simulink model "RadioComm2015"  (Simulink 8.1)
settings: Solver=ode45  StartTime=0.0  StopTime=10.0  RelTol=1e-3
libraries: simulink x6
settings Model: Creator=Brian  LastModifiedBy=Brian
settings DataIOCC: SignalLoggingSaveFormat=Dataset
settings OptimizationCC: ExpressionDepthLimit=128
settings DebuggingCC: FcnCallInpInsideContextMsg=EnableAllAsError
settings GRTTargetCC: CombineOutputUpdateFcns=on  GRTInterface=off

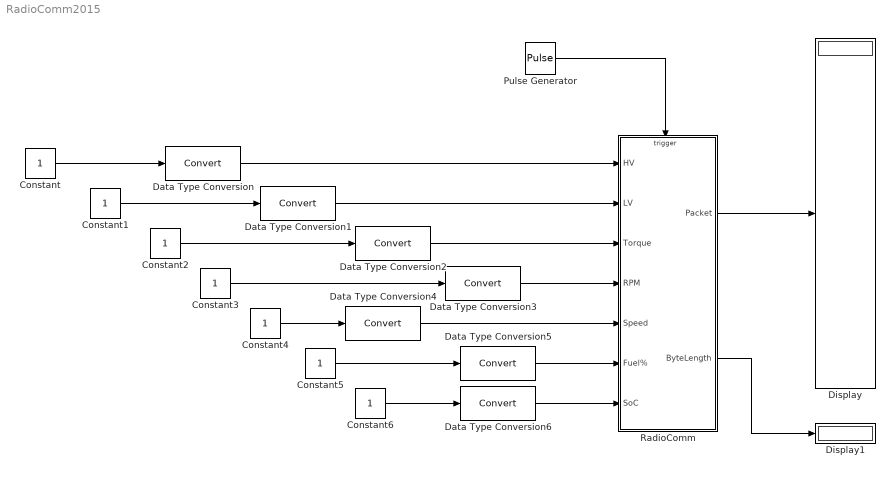
== system RadioComm2015 ==
  Constant{,1..6} (7 alike) : Constant
  Data Type Conversion{,1..6} (7 alike) : DataTypeConversion
  Display : Display
      settings: Format=hex (Stored Integer)
  Display1 : Display
      settings: Format=decimal (Stored Integer)
  Pulse Generator : DiscretePulseGenerator  PulseType=Time based  Period=.5  PulseWidth=5
  RadioComm : Subsystem
  wires:
  Constant/1 -> Data Type Conversion/1
  Constant1/1 -> Data Type Conversion1/1
  Constant2/1 -> Data Type Conversion2/1
  Constant3/1 -> Data Type Conversion3/1
  Constant4/1 -> Data Type Conversion4/1
  Constant5/1 -> Data Type Conversion5/1
  Constant6/1 -> Data Type Conversion6/1
  RadioComm/1(Packet) -> Display/1
  Data Type Conversion/1 -> RadioComm/1(HV)
  Data Type Conversion1/1 -> RadioComm/2(LV)
  Data Type Conversion2/1 -> RadioComm/3(Torque)
  Data Type Conversion3/1 -> RadioComm/4(RPM)
  Data Type Conversion4/1 -> RadioComm/5(Speed)
  Data Type Conversion5/1 -> RadioComm/6(Fuel%)
  Data Type Conversion6/1 -> RadioComm/7(SoC)
  RadioComm/2(ByteLength) -> Display1/1
  Pulse Generator/1 -> RadioComm/Trigger

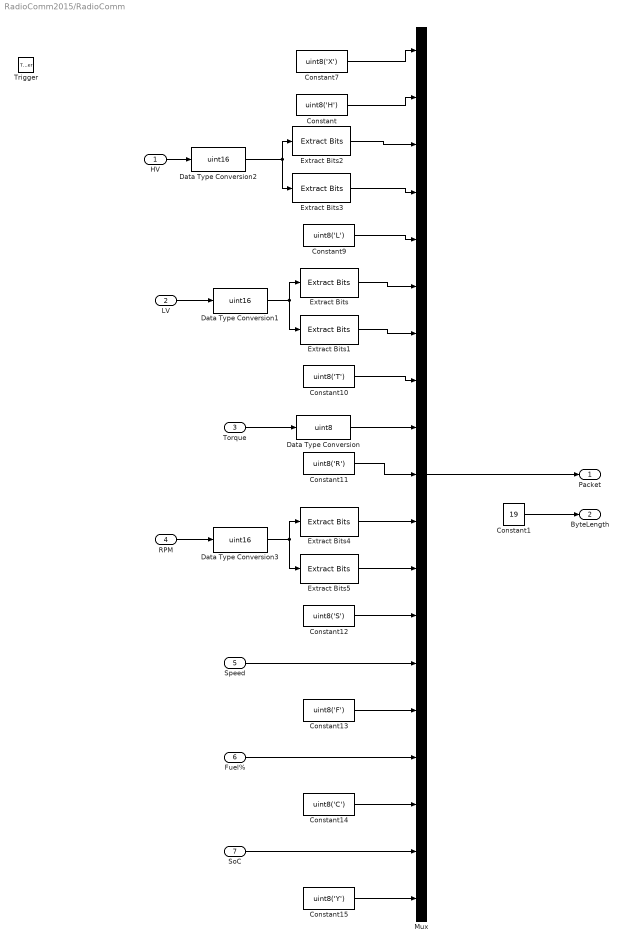
== system RadioComm2015/RadioComm ==
  HV : Inport  OutDataTypeStr=single
  LV : Inport  Port=2  OutDataTypeStr=single
  Torque : Inport  Port=3  OutDataTypeStr=int8
  RPM : Inport  Port=4  OutDataTypeStr=uint16
  Speed : Inport  Port=5  OutDataTypeStr=uint8
  Fuel% : Inport  Port=6  OutDataTypeStr=uint8
  SoC : Inport  Port=7  OutDataTypeStr=uint8
  Trigger : TriggerPort  PortDimensions=1
  Constant : Constant  Value=uint8('H')  OutDataTypeStr=uint8
  Constant1 : Constant  Value=19  OutDataTypeStr=uint8
  Constant10 : Constant  Value=uint8('T')  OutDataTypeStr=uint8
  Constant11 : Constant  Value=uint8('R')  OutDataTypeStr=uint8
  Constant12 : Constant  Value=uint8('S')  OutDataTypeStr=uint8
  Constant13 : Constant  Value=uint8('F')  OutDataTypeStr=uint8
  Constant14 : Constant  Value=uint8('C')  OutDataTypeStr=uint8
  Constant15 : Constant  Value=uint8('Y')  OutDataTypeStr=uint8
  Constant7 : Constant  Value=uint8('X')  OutDataTypeStr=uint8
  Constant9 : Constant  Value=uint8('L')  OutDataTypeStr=uint8
  Data Type Conversion : DataTypeConversion  OutDataTypeStr=uint8  ConvertRealWorld=Stored Integer (SI)  LockScale=on
  Data Type Conversion1 : DataTypeConversion  OutDataTypeStr=uint16  ConvertRealWorld=Stored Integer (SI)  LockScale=on
  Data Type Conversion2 : DataTypeConversion  OutDataTypeStr=uint16  ConvertRealWorld=Stored Integer (SI)  LockScale=on
  Data Type Conversion3 : DataTypeConversion  OutDataTypeStr=uint16  ConvertRealWorld=Stored Integer (SI)  LockScale=on
  Extract Bits : simulink/Logic and Bit Operations/Extract Bits  bitsToExtract=Upper half  numBits=8  bitIdxRange=[0 7]  outScalingMode=Treat bit field as an integer
  Extract Bits1 : simulink/Logic and Bit Operations/Extract Bits  bitsToExtract=Lower half  numBits=8  bitIdxRange=[0 7]  outScalingMode=Treat bit field as an integer
  Extract Bits2 : simulink/Logic and Bit Operations/Extract Bits  bitsToExtract=Upper half  numBits=8  bitIdxRange=[0 7]  outScalingMode=Treat bit field as an integer
  Extract Bits3 : simulink/Logic and Bit Operations/Extract Bits  bitsToExtract=Lower half  numBits=8  bitIdxRange=[0 7]  outScalingMode=Treat bit field as an integer
  Extract Bits4 : simulink/Logic and Bit Operations/Extract Bits  bitsToExtract=Upper half  numBits=8  bitIdxRange=[0 7]  outScalingMode=Treat bit field as an integer
  Extract Bits5 : simulink/Logic and Bit Operations/Extract Bits  bitsToExtract=Lower half  numBits=8  bitIdxRange=[0 7]  outScalingMode=Treat bit field as an integer
  Mux : Mux  Inputs=19
  Packet : Outport
  ByteLength : Outport  Port=2  OutDataTypeStr=uint8
  wires:
  Constant/1 -> Mux/2
  Constant7/1 -> Mux/1
  Mux/1 -> Packet/1
  Data Type Conversion1/1 -> Extract Bits/1, Extract Bits1/1
  LV/1 -> Data Type Conversion1/1
  Data Type Conversion2/1 -> Extract Bits3/1, Extract Bits2/1
  HV/1 -> Data Type Conversion2/1
  Extract Bits2/1 -> Mux/3
  Extract Bits3/1 -> Mux/4
  Constant9/1 -> Mux/5
  Extract Bits/1 -> Mux/6
  Extract Bits1/1 -> Mux/7
  Constant10/1 -> Mux/8
  Torque/1 -> Data Type Conversion/1
  Constant11/1 -> Mux/10
  Data Type Conversion/1 -> Mux/9
  Constant15/1 -> Mux/19
  SoC/1 -> Mux/18
  Constant14/1 -> Mux/17
  Fuel%/1 -> Mux/16
  Constant13/1 -> Mux/15
  Speed/1 -> Mux/14
  Constant12/1 -> Mux/13
  Data Type Conversion3/1 -> Extract Bits5/1, Extract Bits4/1
  RPM/1 -> Data Type Conversion3/1
  Extract Bits4/1 -> Mux/11
  Extract Bits5/1 -> Mux/12
  Constant1/1 -> ByteLength/1
